simulink model "PositionControl"  (R2018b)
settings: Solver=ode3  StartTime=0.0  StopTime=100.0  FixedStep=Ts  RelTol=1e-3
values from neighbouring files (symbols this model uses):
  obsx = 3    [Ejercicio1.m]    (also in Ejercicio2.m = 1)
  obsy = 0    [Ejercicio1.m]    (also in Ejercicio2.m = 2)
  refx = 5    [Ejercicio1.m]
  refy = 0    [Ejercicio1.m]
undefined symbols (not defined in the file or in its folder): DiscIntNeverNeededParam
libraries: fuzblock x1, simulink x1
settings Model: EnablePacing=on  PacingRate=10  Creator=Edu  LastModifiedBy=Edu

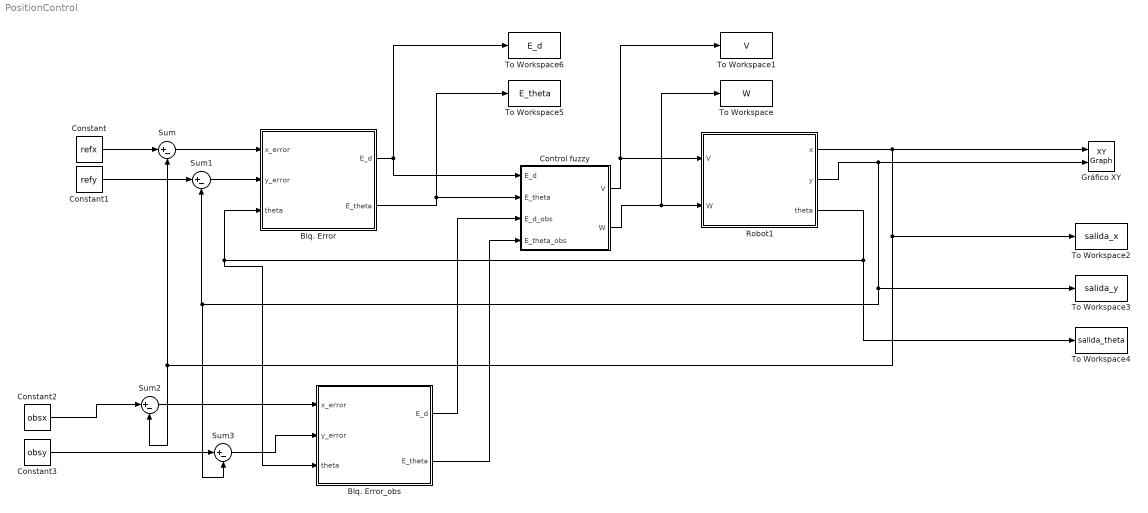
== system PositionControl ==
  Blq. Error : Subsystem
  Blq. Error_obs : Subsystem
  Constant : Constant  Value=refx
  Constant1 : Constant  Value=refy
  Constant2 : Constant  Value=obsx
  Constant3 : Constant  Value=obsy
  Control fuzzy : Subsystem
  Gráfico XY : simulink/Sinks/XY Graph  xmin=0  xmax=10  ymin=-10  ymax=10  st=-1
  Robot1 : Subsystem
  Sum{,1..3} (4 alike) : Sum  Inputs=|+-
  To Workspace : ToWorkspace  VariableName=W  SaveFormat=Structure With Time  SampleTime=-1
  To Workspace1 : ToWorkspace  VariableName=V  SaveFormat=Structure With Time  SampleTime=-1
  To Workspace2 : ToWorkspace  VariableName=salida_x  SaveFormat=Structure With Time  SampleTime=-1
  To Workspace3 : ToWorkspace  VariableName=salida_y  SaveFormat=Structure With Time  SampleTime=-1
  To Workspace4 : ToWorkspace  VariableName=salida_theta  SaveFormat=Structure With Time  SampleTime=-1
  To Workspace5 : ToWorkspace  VariableName=E_theta  SaveFormat=Structure With Time  SampleTime=-1
  To Workspace6 : ToWorkspace  VariableName=E_d  SaveFormat=Structure With Time  SampleTime=-1
  wires:
  Robot1/1(x) -> Gráfico XY/1, To Workspace2/1, Sum/2, Sum2/2
  Robot1/2(y) -> Gráfico XY/2, To Workspace3/1, Sum1/2, Sum3/2
  Robot1/3(theta) -> Blq. Error/3(theta), Blq. Error_obs/3(theta), To Workspace4/1
  Blq. Error/2(E_theta) -> Control fuzzy/2(E_theta), To Workspace5/1
  Blq. Error/1(E_d) -> Control fuzzy/1("E_d "), To Workspace6/1
  Control fuzzy/1(V) -> Robot1/1(V), To Workspace1/1
  Control fuzzy/2("W ") -> Robot1/2(W), To Workspace/1
  Constant/1 -> Sum/1
  Sum/1 -> Blq. Error/1(x_error)
  Constant1/1 -> Sum1/1
  Sum1/1 -> Blq. Error/2(y_error)
  Constant2/1 -> Sum2/1
  Constant3/1 -> Sum3/1
  Sum2/1 -> Blq. Error_obs/1(x_error)
  Sum3/1 -> Blq. Error_obs/2(y_error)
  Blq. Error_obs/1(E_d) -> Control fuzzy/3(E_d_obs)
  Blq. Error_obs/2(E_theta) -> Control fuzzy/4(E_theta_obs)

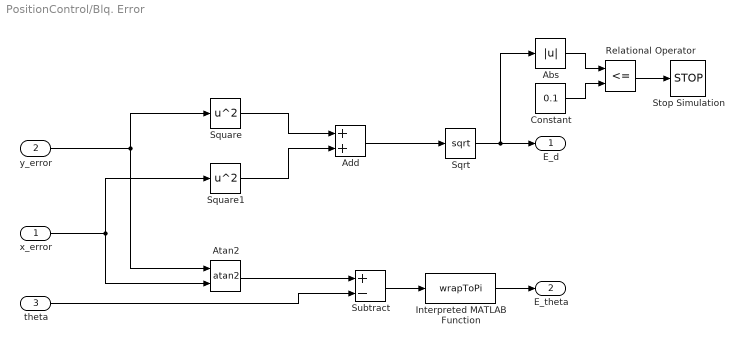
== system PositionControl/Blq. Error ==
  x_error : Inport
  y_error : Inport  Port=2
  theta : Inport  Port=3
  Abs : Abs
  Add : Sum
  Atan2 : Trigonometry  Operator=atan2
  Constant : Constant  Value=0.1
  Interpreted MATLAB Function : MATLABFcn  MATLABFcn=wrapToPi
  Relational Operator : RelationalOperator  Operator=<=  OutDataTypeStr=boolean  RndMeth=Simplest
  Sqrt : Sqrt  SaturateOnIntegerOverflow=on
  Square : Math  Operator=square  SaturateOnIntegerOverflow=on
  Square1 : Math  Operator=square  SaturateOnIntegerOverflow=on
  Stop Simulation : Stop
  Subtract : Sum  Inputs=+-
  E_d : Outport
  E_theta : Outport  Port=2  OutMin=[-pi]  OutMax=[pi]
  wires:
  y_error/1 -> Atan2/1, Square/1
  x_error/1 -> Atan2/2, Square1/1
  Square/1 -> Add/1
  Square1/1 -> Add/2
  Add/1 -> Sqrt/1
  Sqrt/1 -> Abs/1, E_d/1
  Atan2/1 -> Subtract/1
  theta/1 -> Subtract/2
  Abs/1 -> Relational Operator/1
  Constant/1 -> Relational Operator/2
  Relational Operator/1 -> Stop Simulation/1
  Subtract/1 -> Interpreted MATLAB Function/1
  Interpreted MATLAB Function/1 -> E_theta/1

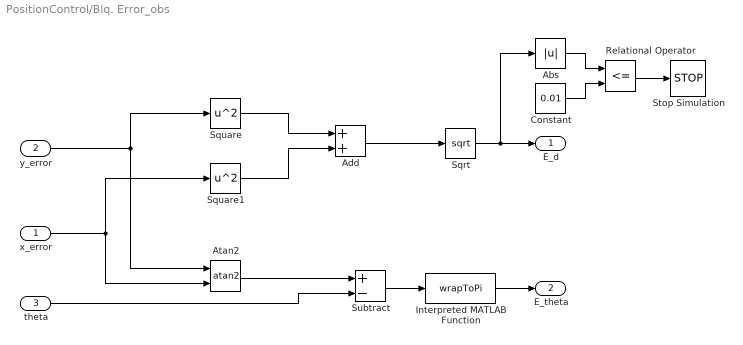
== system PositionControl/Blq. Error_obs ==
  x_error : Inport
  y_error : Inport  Port=2
  theta : Inport  Port=3
  Abs : Abs
  Add : Sum
  Atan2 : Trigonometry  Operator=atan2
  Constant : Constant  Value=0.01
  Interpreted MATLAB Function : MATLABFcn  MATLABFcn=wrapToPi
  Relational Operator : RelationalOperator  Operator=<=  OutDataTypeStr=boolean  RndMeth=Simplest
  Sqrt : Sqrt  SaturateOnIntegerOverflow=on
  Square : Math  Operator=square  SaturateOnIntegerOverflow=on
  Square1 : Math  Operator=square  SaturateOnIntegerOverflow=on
  Stop Simulation : Stop
  Subtract : Sum  Inputs=+-
  E_d : Outport
  E_theta : Outport  Port=2  OutMin=[-pi]  OutMax=[pi]
  wires:
  y_error/1 -> Atan2/1, Square/1
  x_error/1 -> Atan2/2, Square1/1
  Square/1 -> Add/1
  Square1/1 -> Add/2
  Add/1 -> Sqrt/1
  Sqrt/1 -> Abs/1, E_d/1
  Atan2/1 -> Subtract/1
  theta/1 -> Subtract/2
  Abs/1 -> Relational Operator/1
  Constant/1 -> Relational Operator/2
  Relational Operator/1 -> Stop Simulation/1
  Subtract/1 -> Interpreted MATLAB Function/1
  Interpreted MATLAB Function/1 -> E_theta/1

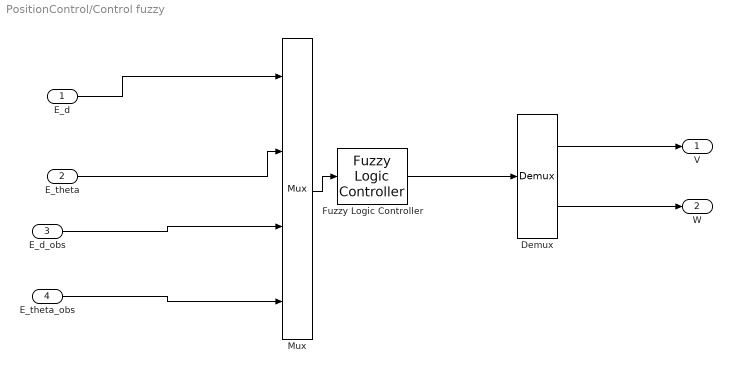
== system PositionControl/Control fuzzy ==
  "E_d " : Inport
  E_theta : Inport  Port=2
  E_d_obs : Inport  Port=3
  E_theta_obs : Inport  Port=4
  Demux : Demux  Outputs=2
  Fuzzy Logic Controller : fuzblock/Fuzzy Logic  Controller  FIS='ControlBorroso.fis'  OutputSampleNumber=101  DataType=double  FuzzifiedInputs=off  RuleFiringStrengths=off  RuleOutputs=off  AggregatedOutputs=off  SimulateUsing=Interpreted execution  OutOfRangeInputValueMessage=warning  NoRuleFiredMessage=warning  EmptyOutputFuzzySetMessage=warning
  Mux : Mux
  V : Outport
  "W " : Outport  Port=2
  wires:
  Mux/1 -> Fuzzy Logic Controller/1
  "E_d "/1 -> Mux/1
  Demux/1 -> V/1
  Demux/2 -> "W "/1
  E_theta/1 -> Mux/2
  Fuzzy Logic Controller/1 -> Demux/1
  E_d_obs/1 -> Mux/3
  E_theta_obs/1 -> Mux/4

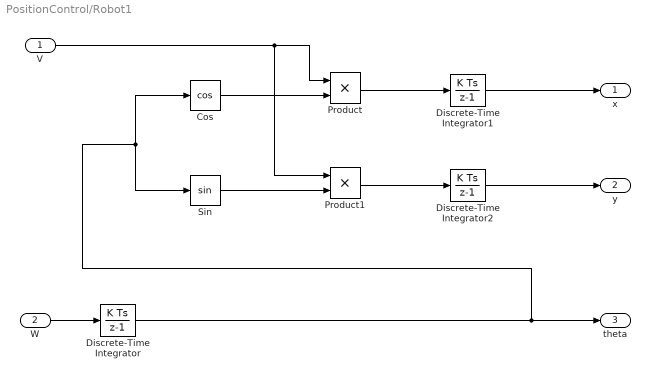
== system PositionControl/Robot1 ==
  V : Inport
  W : Inport  Port=2
  Cos : Trigonometry  Operator=cos
  Discrete-Time Integrator : DiscreteIntegrator  SampleTime=-1  ICPrevOutput=DiscIntNeverNeededParam  ICPrevScaledInput=DiscIntNeverNeededParam
  Discrete-Time Integrator1 : DiscreteIntegrator  SampleTime=-1  ICPrevOutput=DiscIntNeverNeededParam  ICPrevScaledInput=DiscIntNeverNeededParam
  Discrete-Time Integrator2 : DiscreteIntegrator  SampleTime=-1  ICPrevOutput=DiscIntNeverNeededParam  ICPrevScaledInput=DiscIntNeverNeededParam
  Product : Product
  Product1 : Product
  Sin : Trigonometry
  x : Outport
  y : Outport  Port=2
  theta : Outport  Port=3
  wires:
  Sin/1 -> Product1/2
  Product1/1 -> Discrete-Time Integrator2/1
  Product/1 -> Discrete-Time Integrator1/1
  Discrete-Time Integrator2/1 -> y/1
  V/1 -> Product1/1, Product/1
  Discrete-Time Integrator1/1 -> x/1
  Discrete-Time Integrator/1 -> Sin/1, Cos/1, theta/1
  W/1 -> Discrete-Time Integrator/1
  Cos/1 -> Product/2
